simulink model "simulink2"  (R2024a)
settings: Solver=VariableStepAuto  StartTime=0.0  StopTime=100  RelTol=1e-3

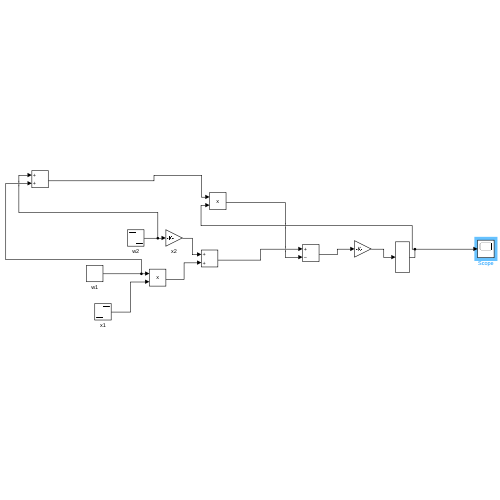
[thumbnail: Simulink's stored preview of the top-level diagram]
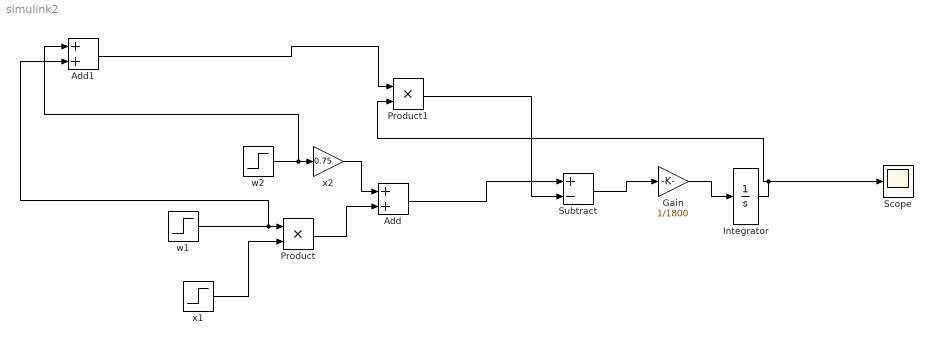
== system simulink2 ==
  Add : Sum
  Add1 : Sum
  Gain : Gain  Gain=1/1800
  Integrator : Integrator  InitialCondition=0.5
  Product : Product
  Product1 : Product
  Scope : Scope
  Subtract : Sum  Inputs=+-
  w1 : Step  Time=0  Before=500  After=400  SampleTime=0
  w2 : Step  Time=15  Before=200  After=100  SampleTime=0
  x1 : Step  Time=15  Before=0.4  After=0.6  SampleTime=0
  x2 : Gain  Gain=0.75
  wires:
  w1/1 -> Add1/2, Product/1
  x1/1 -> Product/2
  w2/1 -> Add1/1, x2/1
  x2/1 -> Add/1
  Product/1 -> Add/2
  Add/1 -> Subtract/1
  Add1/1 -> Product1/1
  Product1/1 -> Subtract/2
  Subtract/1 -> Gain/1
  Gain/1 -> Integrator/1
  Integrator/1 -> Product1/2, Scope/1
